simulink model "pendcartMPC"  (R2020a)
settings: Solver=VariableStepAuto  StartTime=0.0  StopTime=20  MaxStep=1e-3  RelTol=1e-3  EnableMultiTasking=on
undefined symbols (not defined in the file or in its folder): R, sigbuilder_block, Ts, u0
libraries: mympclib x2, simulink_extras x2
settings Model: Creator=The MathWorks, Inc.  LastModifiedBy=kohei
settings SolverCC: AlgebraicLoopSolver=LineSearch
settings DataIOCC: LimitDataPoints=on  SaveFormat=Array  SaveOutput=off  DSMLogging=off  SaveTime=off  ReturnWorkspaceOutputs=off
settings OptimizationCC: LifeSpan=inf
settings DebuggingCC: AlgebraicLoopMsg=none  UnderspecifiedInitializationDetection=Classic  MergeDetectMultiDrivingBlocksExec=none  SolverPrmCheckMsg=warning  AllowSymbolicDim=off  StateNameClashWarn=warning  SFUnexpectedBacktrackingDiag=warning  SFNoUnconditionalDefaultTransitionDiag=warning  SFExecutionAtInitializationDiag=none  ArithmeticOperatorsInVariantConditions=warning
settings HardwareCC: ProdBitPerPointer=32  ProdBitPerSizeT=32  ProdBitPerPtrDiffT=32  ProdLargestAtomicFloat=None  ProdIntDivRoundTo=Undefined  ProdEndianess=Unspecified  ProdWordSize=32  ProdHWDeviceType=32-bit Generic
settings ModelReferenceCC: PropagateSignalLabelsOutOfModel=off
settings SFSimCC: SimUseLocalCustomCode=off  CustomCodeUndefinedFunction=UseInterfaceOnly
settings RTWCC: RTWUseLocalCustomCode=off
settings CodeAppCC: StateflowObjectComments=on
settings GRTTargetCC: TargetLangStandard=C89/C90 (ANSI)
settings ConfigComp: CovMetricSettings=dw  CovHtmlReporting=on  CovSaveCumulativeToWorkspaceVar=on  CovSaveSingleToWorkspaceVar=on  CovExternalEMLEnable=off  CovSFcnEnable=off
settings SimscapeCC: SimscapeNormalizeSystem=off  SimscapeNominalValues="[{\"value\":\"10\",\"unit\":\"V\"},{\"value\":\"1\",\"unit\":\"A\"},{\"value\":\"10\",\"unit\":\"N*m\"},{\"value\":\"10\",\"unit\":\"bar\"},{\"value\":\"100\",\"unit\":\"kJ/kg\"},{\"value\":\"1\",\"unit\":\"kW\"},{\"value\":\"300\",\"unit\":\"K\"},{\"value\":\"100\",\"unit\":\"cm^3/s\"},{\"value\":\"1\",\"unit\":\"kN\"},{\"value\":\"1\",\"unit\":\"g/cm^3\"},{\"value\":\"1\",\"unit\":\"l\"},{\"value\":\"1\",\"unit\":\"cm^2\"},{\"value\":\"60\",\"unit\":\"Hz\"}]"
settings ConfigurationSet: Description=SimMechanics 2G
settings ExplorerConfigSet: InternalSimMechanicsExplorerSettings="<ExplorerConfiguration><canonicalview>default</canonicalview><AnimationSetting><BasePlaybackSpeed>1.0</BasePlaybackSpeed><PlaybackSpeedFactor>1.0</PlaybackSpeedFactor></AnimationSetting><TilePanel><TileInfo><Tiles Columns=\"1\" Count=\"1\" Rows=\"1\"><Column Left=\"2\" Weight=\"1\"/><Column Left=\"1552\"/><Row Top=\"2\" Weight=\"1\"/><Row Top=\"932\"/><Tile Height=\"1\" Width=\"1\" X=\"0\" Y=\"0\"/></Tiles></TileInfo><SceneInfo><SceneViewer><BGColor><R>0.60000002384185791</R><G>0.60000002384185791</G><B>0.60000002384185791</B></BGColor><Camera><Position><X>0.027865189060748197</X><Y>-2.5719092456962986</Y><Z>0.23157896538506753</Z></Position><Center><X>0.62659712312732463</X><Y>-0.46110119691712204</Y><Z>0.22087365386473376</Z></Center><Up><X>-0.0079438354874226333</X><Y>0.0073246425924307582</Y><Z>0.99994162084025784</Z></Up><Left>-0.24533778208815546</Left><Right>0.24533778208815546</Right><Bottom>-0.79734779727023208</Bottom><Top>0.79734779727023208</Top></Camera></SceneViewer></SceneInfo></TilePanel></ExplorerConfiguration>"

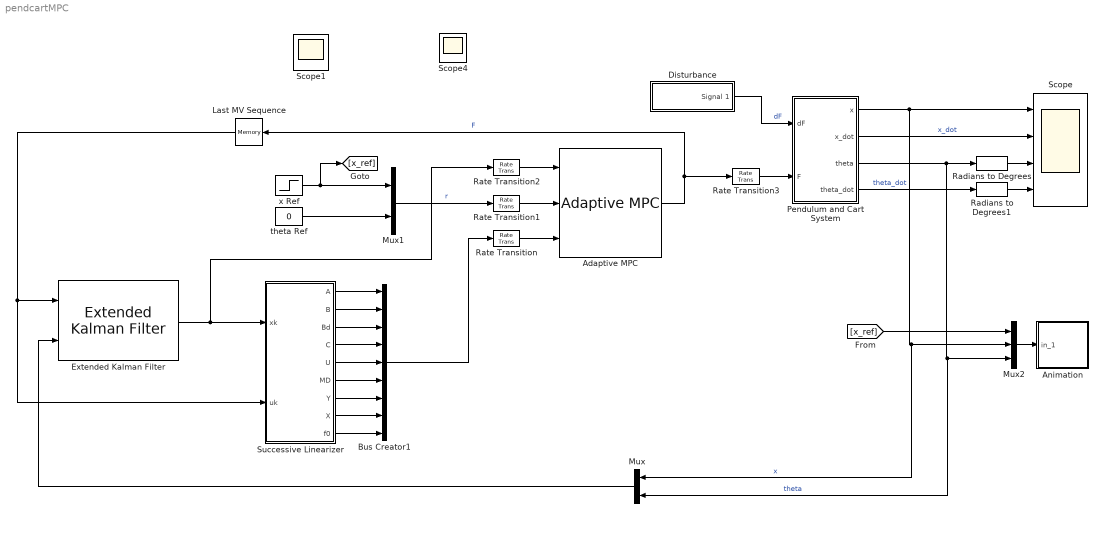
== system pendcartMPC ==
  Adaptive MPC : mympclib/Adaptive MPC  params=params  numState=4  numRef=2  numMV=1  Ts=Ts  enableDist=off  numDist=1  enableSlack=off  enableStatus=off  enableMVseq=off
      settings: SourceProductName=My MPC Library
  Animation : Subsystem  mask(Pendulum plot){RefBlock=x Ref}
      mask prompts: RefBlock "Cart Reference Signal Block Name:"
      mask help: Pendulum plot
      mask Help: Pendulum animation function using Handle graphics.
      mask Display: plot([-10 10],[0 0],[-2 -2 2 2],[0 1 1 0],[0 3],[1 5])
  Bus Creator1 : BusCreator  Inputs=9  OutDataTypeStr=Bus: sysBus
  Disturbance : Subsystem  Tag=STV Subsys  LoadFcn=sigbuilder_block('load');  StartFcn=sigbuilder_block('start');  StopFcn=sigbuilder_block('stop');  ClipboardFcn=sigbuilder_block('clipboard');  mask(Sigbuilder block){tuvar=[0:10]}
      mask help: Simulink:masks:SigbuilderBlock_MD
      mask init:
      | if ~strcmp(get_param(bdroot(gcbh),'SimulationStatus'),'stopped') tuvar = sigbuilder_block('maskInit'); end
      settings: CopyFcn=sigbuilder_block('copy');  DeleteFcn=sigbuilder_block('delete');  ModelCloseFcn=sigbuilder_block('modelClose');  PreSaveFcn=sigbuilder_block('preSave');  PauseFcn=sigbuilder_block('pause');  ContinueFcn=sigbuilder_block('continue');  NameChangeFcn=sigbuilder_block('namechange');  OpenFcn=sigbuilder_block('open',[402.828 122.5 551.172 357.5 ]);  CloseFcn=sigbuilder_block('close');
      mask Display: plot(0, 0, 100, 100,[2, 2, 32, 32, 2], [68, 8, 8, 68, 68],[32, 2], [38, 38], [32, 19, 2],[53, 60, 44], [32, 17, 17, 2],[16, 16, 31, 31]);txt = getActiveGroup(gcbh);text(2, 100, txt,'verticalAlignment', 'top');
  Extended Kalman Filter : mympclib/Extended Kalman Filter  stateFunction='stateFcn'  jacobianStateFunction='jacobianStateFcn'  measurementFunction='measuermentFcn'  jacobianMeasurmentFunction='jacobianMeasurementFcn'  Bv=Bv  Q=Q  R=R  xhat0=xhat0  P0=P0  Ts=Ts  numState=n  numOutput=l  enableP=off  enableG=off
      settings: SourceProductName=My MPC Library
  Last MV Sequence : Memory  InitialCondition=u0  InheritSampleTime=on
  Mux : Mux  Inputs=2
  Mux1 : Mux  Inputs=2
  Mux2 : Mux  Inputs=3
  Pendulum and Cart System : Subsystem  mask{mCartPara=1, mPendPara=1, gPara=9.81, LPara=0.5, KdPara=10}
      mask prompts: mCartPara "Mass of Cart"; mPendPara "Mass of Pendulum"; gPara "Gravity"; LPara "Length of Pendulum"; KdPara "Friction coefficient of Cart"
      mask help: Pendulum and Cart System
      mask init:
      | mCart = str2double(get_param(gcb,'mCartPara'));
      | mPend = str2double(get_param(gcb,'mPendPara'));
      | g = str2double(get_param(gcb,'gPara'));
      | L = str2double(get_param(gcb,'LPara'));
      | Kd = str2double(get_param(gcb,'KdPara'));
  Radians to Degrees : simulink_extras/Transformations/Radians to Degrees
  Radians to Degrees1 : simulink_extras/Transformations/Radians to Degrees
  Rate Transition{,1..3} (4 alike) : RateTransition
  Scope : Scope  NumInputPorts=4
  Successive Linearizer : MATLAB Function  TreatAsAtomicUnit=on
  theta Ref : Constant  Value=0
  x Ref : Step  After=20  SampleTime=Ts
  Scope1 : Scope
  Scope4 : Scope
  wires:
  Pendulum and Cart System/4(theta_dot) -> Radians to Degrees1/1  "theta_dot"
  Pendulum and Cart System/3(theta) -> Radians to Degrees/1, Mux/2, Mux2/3  "theta"
  Pendulum and Cart System/2(x_dot) -> Scope/2  "x_dot"
  Pendulum and Cart System/1(x) -> Scope/1, Mux/1, Mux2/2  "x"
  Disturbance/1(Signal 1) -> Pendulum and Cart System/1(dF)  "dF"
  Last MV Sequence/1 -> Successive Linearizer/2(uk), Extended Kalman Filter/1
  Adaptive MPC/1 -> Last MV Sequence/1, Rate Transition3/1  "F"
  Bus Creator1/1 -> Rate Transition/1
  Mux1/1 -> Rate Transition1/1  "r"
  Rate Transition/1 -> Adaptive MPC/3
  Rate Transition1/1 -> Adaptive MPC/2
  Rate Transition2/1 -> Adaptive MPC/1
  theta Ref/1 -> Mux1/2
  Rate Transition3/1 -> Pendulum and Cart System/2(F)
  Mux2/1 -> Animation/1(in_1)
  [x_ref] -> Mux2/1
  x Ref/1 -> [x_ref], Mux1/1
  Radians to Degrees/1 -> Scope/3
  Radians to Degrees1/1 -> Scope/4
  Successive Linearizer/1(A) -> Bus Creator1/1
  Successive Linearizer/2(B) -> Bus Creator1/2
  Successive Linearizer/3(Bd) -> Bus Creator1/3
  Successive Linearizer/4(C) -> Bus Creator1/4
  Successive Linearizer/5(U) -> Bus Creator1/5
  Successive Linearizer/6(MD) -> Bus Creator1/6
  Successive Linearizer/7(Y) -> Bus Creator1/7
  Successive Linearizer/8(X) -> Bus Creator1/8
  Successive Linearizer/9(f0) -> Bus Creator1/9
  Extended Kalman Filter/1 -> Rate Transition2/1, Successive Linearizer/1(xk)
  Mux/1 -> Extended Kalman Filter/2

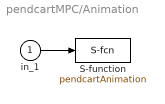
== system pendcartMPC/Animation ==
  in_1 : Inport
  S-function : S-Function  FunctionName=pendcartAnimation  Parameters=RefBlock  SFunctionDeploymentMode=off  EnableBusSupport=off
      settings: DeleteFcn=pendcartAnimation([],[],[],'DeleteBlock');
  wires:
  in_1/1 -> S-function/1

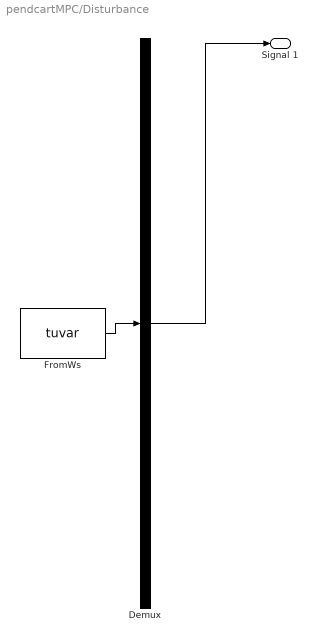
== system pendcartMPC/Disturbance ==
  Demux : Demux  Tag=STV Demux  Outputs=1
      settings: DisplayOption=none
  FromWs : FromWorkspace  Tag=STV FromWs  VariableName=tuvar
      SigBuilderData=|
      | common.afterFinalStr = 'Extrapolate'
      | common.sampleTime = 0
      | dataSet.timeRange = [0 20]
      | dataSet.name = 'Group 1'
      | sbobj.Groups.Name = 'Group 1'
      | sbobj.Groups.Signals.Name = 'Signal 1'
      | sbobj.Groups.Signals.XData = [0 10 10.5 11 20]
      | sbobj.Groups.Signals.YData = [0 0 4 0 0]
      | sbobj.Groups.TimeRange = [0 20]
  Signal 1 : Outport  Tag=STV Outport  VectorParamsAs1DForOutWhenUnconnected=off
  wires:
  FromWs/1 -> Demux/1
  Demux/1 -> Signal 1/1

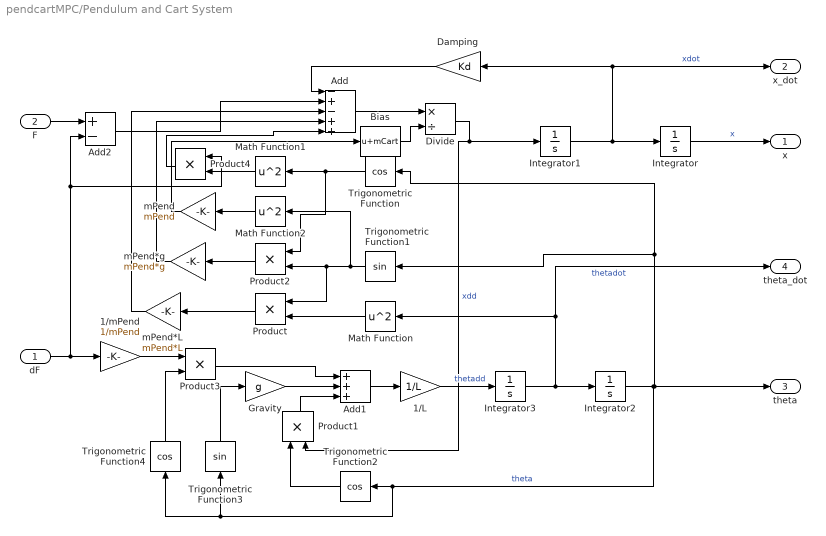
== system pendcartMPC/Pendulum and Cart System ==
  dF : Inport
  F : Inport  Port=2
  1/L : Gain  Gain=1/L
  1/mPend : Gain  Gain=1/mPend
  Add : Sum  Inputs=-+-++
  Add1 : Sum  Inputs=+++
  Add2 : Sum  Inputs=+-
  Bias : Bias  Bias=mCart
  Damping : Gain  Gain=Kd
  Divide : Product  Inputs=*/
  Gravity : Gain  Gain=g
  Integrator : Integrator  ContinuousStateAttributes='x'
  Integrator1 : Integrator  ContinuousStateAttributes='xdot'
  Integrator2 : Integrator  ContinuousStateAttributes='theta'
  Integrator3 : Integrator  ContinuousStateAttributes='thetadot'
  Math Function : Math  Operator=square  SignedPower=on  SaturateOnIntegerOverflow=on
  Math Function1 : Math  Operator=square  SignedPower=on  SaturateOnIntegerOverflow=on
  Math Function2 : Math  Operator=square  SignedPower=on  SaturateOnIntegerOverflow=on
  Product{,1..4} (5 alike) : Product
  Trigonometric Function : Trigonometry  Operator=cos
  Trigonometric Function1 : Trigonometry
  Trigonometric Function2 : Trigonometry  Operator=cos
  Trigonometric Function3 : Trigonometry
  Trigonometric Function4 : Trigonometry  Operator=cos
  mPend : Gain  Gain=mPend
  mPend*L : Gain  Gain=mPend*L
  mPend*g : Gain  Gain=mPend*g
  x : Outport  VectorParamsAs1DForOutWhenUnconnected=off
  x_dot : Outport  Port=2  VectorParamsAs1DForOutWhenUnconnected=off
  theta : Outport  Port=3  VectorParamsAs1DForOutWhenUnconnected=off
  theta_dot : Outport  Port=4  VectorParamsAs1DForOutWhenUnconnected=off
  wires:
  mPend/1 -> Bias/1
  Bias/1 -> Divide/2
  Math Function2/1 -> mPend/1
  Product4/1 -> Add/5
  Math Function1/1 -> Product4/2
  mPend*g/1 -> Add/4
  Product1/1 -> Add1/3
  Math Function/1 -> Product/2
  1/L/1 -> Integrator3/1  "thetadd"
  dF/1 -> 1/mPend/1, Product4/1, Add2/2
  1/mPend/1 -> Product3/1
  Trigonometric Function4/1 -> Product3/2
  Damping/1 -> Add/1
  F/1 -> Add2/1
  Trigonometric Function3/1 -> Gravity/1
  Gravity/1 -> Add1/2
  Trigonometric Function/1 -> Math Function1/1, Product2/1
  Integrator3/1 -> Integrator2/1, Math Function/1, theta_dot/1  "thetadot"
  Integrator2/1 -> Trigonometric Function2/1, Trigonometric Function3/1, Trigonometric Function4/1, Trigonometric Function1/1, Trigonometric Function/1, theta/1  "theta"
  Product3/1 -> Add1/1
  Add/1 -> Divide/1
  Divide/1 -> Integrator1/1, Product1/2  "xdd"
  Trigonometric Function2/1 -> Product1/1
  Trigonometric Function1/1 -> Math Function2/1, Product/1, Product2/2
  Integrator/1 -> x/1  "x"
  Integrator1/1 -> Damping/1, x_dot/1, Integrator/1  "xdot"
  Product2/1 -> mPend*g/1
  Add1/1 -> 1/L/1
  Add2/1 -> Add/2
  mPend*L/1 -> Add/3
  Product/1 -> mPend*L/1

== matlab function pendcartMPC/Successive Linearizer ==
  settings: updateMethod=DISCRETE  sampleTime=Ts
  data: xk input; uk input; A output; B output; Bd output; C output; U output; MD output; Y output; X output; f0 output; Ts parameter
function [A,B,Bd,C,U,MD,Y,X,f0] = fcn(xk,uk,Ts)
% analytical linearization (continuous time)
n = length(xk);
m = length(uk);
Ac = zeros(n);
Bc = zeros(n,m);
Bdc = zeros(n,1);
Cc = zeros(2,n);
U = zeros(m,1);
MD = 0;
Y = zeros(2,1);
X = zeros(n,1);
f0 = zeros(n,1);
[Ac,Bc,Bdc,Cc,U,MD,Y,X,f0c] = mypendulumCT(xk, uk);

% obtain matrices
A = eye(n)+Ts*Ac; %Euler approximation
B = Ts*Bc;
Bd = Ts*Bdc;
C = Cc;
f0 = Ts*f0c;
end
